simulink library "Course_Holes_Lib"  (R2026a)
settings: Solver=ode45  EnableMultiTasking=on
undefined symbols (not defined in the file): Mini_Golf_Param, X, Y, Z
libraries: Golf_Components_Lib x67, Contact_Forces_Lib x18, sm_lib x12
(part 2 of 2)

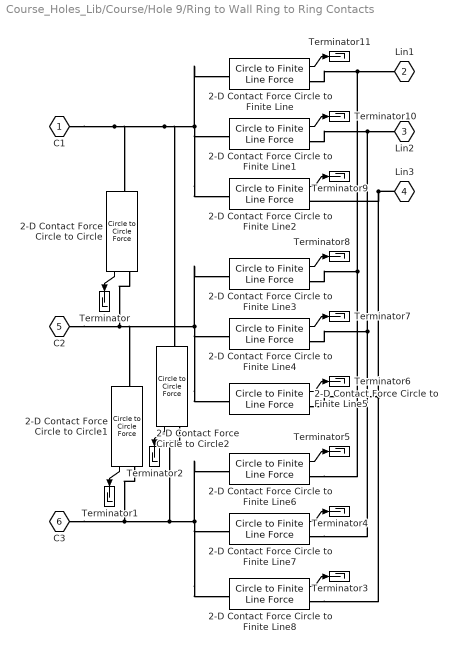
== system Course_Holes_Lib/Course/Hole 9/Ring to Wall Ring to Ring Contacts ==
  2-D Contact Force Circle to Circle : Contact_Forces_Lib/2D/Circle to Circle Force  cirB_rad=Mini_Golf_Param.Hole_9.Extr1.Ring_Outer_Diameter/2  cirF_rad=Mini_Golf_Param.Hole_9.Extr2.Ring_Outer_Diameter/2  active_angle=[-180 180]  force_law=Linear  k_contact=Mini_Golf_Param.Wall.Stiffness  b_contact=Mini_Golf_Param.Wall.Damping  pen_full_damp_F=1e-4  pen_exponent=1  custom_param_1=1  custom_param_2=1  friction_law=None  mu_kinetic=0.5  mu_static=0.7  v_thr=0.001  vis_on=off  vis_opc_en=0  vis_len_cirBz=0.1  vis_len_cirBx=0.005  vis_len_cirFz=0.1  vis_len_cirFx=0.005  vis_clr=[0.9 0.2 0.2]  vis_opc=0.7
      settings: SourceProductName=Simscape Multibody Contact Forces Library
  2-D Contact Force Circle to Circle1 : Contact_Forces_Lib/2D/Circle to Circle Force  cirB_rad=Mini_Golf_Param.Hole_9.Extr3.Ring_Outer_Diameter/2  cirF_rad=Mini_Golf_Param.Hole_9.Extr2.Ring_Outer_Diameter/2  active_angle=[-180 180]  force_law=Linear  k_contact=Mini_Golf_Param.Wall.Stiffness  b_contact=Mini_Golf_Param.Wall.Damping  pen_full_damp_F=1e-4  pen_exponent=1  custom_param_1=1  custom_param_2=1  friction_law=None  mu_kinetic=0.5  mu_static=0.7  v_thr=0.001  vis_on=off  vis_opc_en=0  vis_len_cirBz=0.1  vis_len_cirBx=0.005  vis_len_cirFz=0.1  vis_len_cirFx=0.005  vis_clr=[0.9 0.2 0.2]  vis_opc=0.7
      settings: SourceProductName=Simscape Multibody Contact Forces Library
  2-D Contact Force Circle to Circle2 : Contact_Forces_Lib/2D/Circle to Circle Force  cirB_rad=Mini_Golf_Param.Hole_9.Extr3.Ring_Outer_Diameter/2  cirF_rad=Mini_Golf_Param.Hole_9.Extr1.Ring_Outer_Diameter/2  active_angle=[-180 180]  force_law=Linear  k_contact=Mini_Golf_Param.Wall.Stiffness  b_contact=Mini_Golf_Param.Wall.Damping  pen_full_damp_F=1e-4  pen_exponent=1  custom_param_1=1  custom_param_2=1  friction_law=None  mu_kinetic=0.5  mu_static=0.7  v_thr=0.001  vis_on=off  vis_opc_en=0  vis_len_cirBz=0.1  vis_len_cirBx=0.005  vis_len_cirFz=0.1  vis_len_cirFx=0.005  vis_clr=[0.9 0.2 0.2]  vis_opc=0.7
      settings: SourceProductName=Simscape Multibody Contact Forces Library
  2-D Contact Force Circle to Finite Line : Contact_Forces_Lib/2D/Circle to Finite Line Force  circle_rad=Mini_Golf_Param.Hole_9.Extr1.Ring_Outer_Diameter/2  line_depth=Mini_Golf_Param.Wall.Width/2  line_length=Mini_Golf_Param.Hole_9.Wall_Right.Length  force_law=Linear  k_contact=Mini_Golf_Param.Wall.Stiffness  b_contact=Mini_Golf_Param.Wall.Damping  pen_full_damp_F=1e-4  pen_exponent=1  custom_param_1=1  custom_param_2=1  friction_law=None  mu_kinetic=0.5  mu_static=0.7  v_thr=0.001  vis_on=off  vis_opc_en=0  vis_len_linBz=0.1  vis_len_linBx=0.005  vis_len_cirFz=0.1  vis_len_cirFx=0.005  vis_clr=[0.9 0.2 0.2]  vis_opc=0.7
      settings: SourceProductName=Simscape Multibody Contact Forces Library
  2-D Contact Force Circle to Finite Line1 : Contact_Forces_Lib/2D/Circle to Finite Line Force  circle_rad=Mini_Golf_Param.Hole_9.Extr1.Ring_Outer_Diameter/2  line_depth=Mini_Golf_Param.Wall.Width/2  line_length=Mini_Golf_Param.Hole_9.Wall_Back.Length  force_law=Linear  k_contact=Mini_Golf_Param.Wall.Stiffness  b_contact=Mini_Golf_Param.Wall.Damping  pen_full_damp_F=1e-4  pen_exponent=1  custom_param_1=1  custom_param_2=1  friction_law=None  mu_kinetic=0.5  mu_static=0.7  v_thr=0.001  vis_on=off  vis_opc_en=0  vis_len_linBz=0.1  vis_len_linBx=0.005  vis_len_cirFz=0.1  vis_len_cirFx=0.005  vis_clr=[0.9 0.2 0.2]  vis_opc=0.7
      settings: SourceProductName=Simscape Multibody Contact Forces Library
  2-D Contact Force Circle to Finite Line2 : Contact_Forces_Lib/2D/Circle to Finite Line Force  circle_rad=Mini_Golf_Param.Hole_9.Extr1.Ring_Outer_Diameter/2  line_depth=Mini_Golf_Param.Wall.Width/2  line_length=Mini_Golf_Param.Hole_9.Wall_Right.Length  force_law=Linear  k_contact=Mini_Golf_Param.Wall.Stiffness  b_contact=Mini_Golf_Param.Wall.Damping  pen_full_damp_F=1e-4  pen_exponent=1  custom_param_1=1  custom_param_2=1  friction_law=None  mu_kinetic=0.5  mu_static=0.7  v_thr=0.001  vis_on=off  vis_opc_en=0  vis_len_linBz=0.1  vis_len_linBx=0.005  vis_len_cirFz=0.1  vis_len_cirFx=0.005  vis_clr=[0.9 0.2 0.2]  vis_opc=0.7
      settings: SourceProductName=Simscape Multibody Contact Forces Library
  2-D Contact Force Circle to Finite Line3 : Contact_Forces_Lib/2D/Circle to Finite Line Force  circle_rad=Mini_Golf_Param.Hole_9.Extr2.Ring_Outer_Diameter/2  line_depth=Mini_Golf_Param.Wall.Width/2  line_length=Mini_Golf_Param.Hole_9.Wall_Right.Length  force_law=Linear  k_contact=Mini_Golf_Param.Wall.Stiffness  b_contact=Mini_Golf_Param.Wall.Damping  pen_full_damp_F=1e-4  pen_exponent=1  custom_param_1=1  custom_param_2=1  friction_law=None  mu_kinetic=0.5  mu_static=0.7  v_thr=0.001  vis_on=off  vis_opc_en=0  vis_len_linBz=0.1  vis_len_linBx=0.005  vis_len_cirFz=0.1  vis_len_cirFx=0.005  vis_clr=[0.9 0.2 0.2]  vis_opc=0.7
      settings: SourceProductName=Simscape Multibody Contact Forces Library
  2-D Contact Force Circle to Finite Line4 : Contact_Forces_Lib/2D/Circle to Finite Line Force  circle_rad=Mini_Golf_Param.Hole_9.Extr2.Ring_Outer_Diameter/2  line_depth=Mini_Golf_Param.Wall.Width/2  line_length=Mini_Golf_Param.Hole_9.Wall_Back.Length  force_law=Linear  k_contact=Mini_Golf_Param.Wall.Stiffness  b_contact=Mini_Golf_Param.Wall.Damping  pen_full_damp_F=1e-4  pen_exponent=1  custom_param_1=1  custom_param_2=1  friction_law=None  mu_kinetic=0.5  mu_static=0.7  v_thr=0.001  vis_on=off  vis_opc_en=0  vis_len_linBz=0.1  vis_len_linBx=0.005  vis_len_cirFz=0.1  vis_len_cirFx=0.005  vis_clr=[0.9 0.2 0.2]  vis_opc=0.7
      settings: SourceProductName=Simscape Multibody Contact Forces Library
  2-D Contact Force Circle to Finite Line5 : Contact_Forces_Lib/2D/Circle to Finite Line Force  circle_rad=Mini_Golf_Param.Hole_9.Extr2.Ring_Outer_Diameter/2  line_depth=Mini_Golf_Param.Wall.Width/2  line_length=Mini_Golf_Param.Hole_9.Wall_Right.Length  force_law=Linear  k_contact=Mini_Golf_Param.Wall.Stiffness  b_contact=Mini_Golf_Param.Wall.Damping  pen_full_damp_F=1e-4  pen_exponent=1  custom_param_1=1  custom_param_2=1  friction_law=None  mu_kinetic=0.5  mu_static=0.7  v_thr=0.001  vis_on=off  vis_opc_en=0  vis_len_linBz=0.1  vis_len_linBx=0.005  vis_len_cirFz=0.1  vis_len_cirFx=0.005  vis_clr=[0.9 0.2 0.2]  vis_opc=0.7
      settings: SourceProductName=Simscape Multibody Contact Forces Library
  2-D Contact Force Circle to Finite Line6 : Contact_Forces_Lib/2D/Circle to Finite Line Force  circle_rad=Mini_Golf_Param.Hole_9.Extr3.Ring_Outer_Diameter/2  line_depth=Mini_Golf_Param.Wall.Width/2  line_length=Mini_Golf_Param.Hole_9.Wall_Right.Length  force_law=Linear  k_contact=Mini_Golf_Param.Wall.Stiffness  b_contact=Mini_Golf_Param.Wall.Damping  pen_full_damp_F=1e-4  pen_exponent=1  custom_param_1=1  custom_param_2=1  friction_law=None  mu_kinetic=0.5  mu_static=0.7  v_thr=0.001  vis_on=off  vis_opc_en=0  vis_len_linBz=0.1  vis_len_linBx=0.005  vis_len_cirFz=0.1  vis_len_cirFx=0.005  vis_clr=[0.9 0.2 0.2]  vis_opc=0.7
      settings: SourceProductName=Simscape Multibody Contact Forces Library
  2-D Contact Force Circle to Finite Line7 : Contact_Forces_Lib/2D/Circle to Finite Line Force  circle_rad=Mini_Golf_Param.Hole_9.Extr3.Ring_Outer_Diameter/2  line_depth=Mini_Golf_Param.Wall.Width/2  line_length=Mini_Golf_Param.Hole_9.Wall_Back.Length  force_law=Linear  k_contact=Mini_Golf_Param.Wall.Stiffness  b_contact=Mini_Golf_Param.Wall.Damping  pen_full_damp_F=1e-4  pen_exponent=1  custom_param_1=1  custom_param_2=1  friction_law=None  mu_kinetic=0.5  mu_static=0.7  v_thr=0.001  vis_on=off  vis_opc_en=0  vis_len_linBz=0.1  vis_len_linBx=0.005  vis_len_cirFz=0.1  vis_len_cirFx=0.005  vis_clr=[0.9 0.2 0.2]  vis_opc=0.7
      settings: SourceProductName=Simscape Multibody Contact Forces Library
  2-D Contact Force Circle to Finite Line8 : Contact_Forces_Lib/2D/Circle to Finite Line Force  circle_rad=Mini_Golf_Param.Hole_9.Extr3.Ring_Outer_Diameter/2  line_depth=Mini_Golf_Param.Wall.Width/2  line_length=Mini_Golf_Param.Hole_9.Wall_Right.Length  force_law=Linear  k_contact=Mini_Golf_Param.Wall.Stiffness  b_contact=Mini_Golf_Param.Wall.Damping  pen_full_damp_F=1e-4  pen_exponent=1  custom_param_1=1  custom_param_2=1  friction_law=None  mu_kinetic=0.5  mu_static=0.7  v_thr=0.001  vis_on=off  vis_opc_en=0  vis_len_linBz=0.1  vis_len_linBx=0.005  vis_len_cirFz=0.1  vis_len_cirFx=0.005  vis_clr=[0.9 0.2 0.2]  vis_opc=0.7
      settings: SourceProductName=Simscape Multibody Contact Forces Library
  Terminator{,1..11} (12 alike) : Terminator
  C1 : PMIOPort  Side=Left
  Lin1 : PMIOPort  Port=2  Side=Right
  Lin2 : PMIOPort  Port=3  Side=Right
  Lin3 : PMIOPort  Port=4  Side=Right
  C2 : PMIOPort  Port=5  Side=Left
  C3 : PMIOPort  Port=6  Side=Left
  wires:
  2-D Contact Force Circle to Circle/1 -> Terminator/1
  2-D Contact Force Circle to Circle1/1 -> Terminator1/1
  2-D Contact Force Circle to Circle2/1 -> Terminator2/1
  2-D Contact Force Circle to Finite Line8/1 -> Terminator3/1
  2-D Contact Force Circle to Finite Line7/1 -> Terminator4/1
  2-D Contact Force Circle to Finite Line6/1 -> Terminator5/1
  2-D Contact Force Circle to Finite Line5/1 -> Terminator6/1
  2-D Contact Force Circle to Finite Line4/1 -> Terminator7/1
  2-D Contact Force Circle to Finite Line3/1 -> Terminator8/1
  2-D Contact Force Circle to Finite Line2/1 -> Terminator9/1
  2-D Contact Force Circle to Finite Line1/1 -> Terminator10/1
  2-D Contact Force Circle to Finite Line/1 -> Terminator11/1
  connections:
  2-D Contact Force Circle to Finite Line5/RConn1 -- 2-D Contact Force Circle to Finite Line8/RConn1 -- 2-D Contact Force Circle to Finite Line2/RConn1 -- Lin3/RConn1
  2-D Contact Force Circle to Finite Line4/RConn1 -- 2-D Contact Force Circle to Finite Line7/RConn1 -- 2-D Contact Force Circle to Finite Line1/RConn1 -- Lin2/RConn1
  2-D Contact Force Circle to Finite Line3/RConn1 -- 2-D Contact Force Circle to Finite Line6/RConn1 -- 2-D Contact Force Circle to Finite Line/RConn1 -- Lin1/RConn1
  C1/RConn1 -- 2-D Contact Force Circle to Circle/LConn1 -- 2-D Contact Force Circle to Circle2/LConn1 -- 2-D Contact Force Circle to Finite Line2/LConn1 -- 2-D Contact Force Circle to Finite Line1/LConn1 -- 2-D Contact Force Circle to Finite Line/LConn1
  C2/RConn1 -- 2-D Contact Force Circle to Circle1/LConn1 -- 2-D Contact Force Circle to Finite Line3/LConn1 -- 2-D Contact Force Circle to Finite Line4/LConn1 -- 2-D Contact Force Circle to Finite Line5/LConn1 -- 2-D Contact Force Circle to Circle/RConn1
  C3/RConn1 -- 2-D Contact Force Circle to Circle1/RConn1 -- 2-D Contact Force Circle to Circle2/RConn1 -- 2-D Contact Force Circle to Finite Line6/LConn1 -- 2-D Contact Force Circle to Finite Line7/LConn1 -- 2-D Contact Force Circle to Finite Line8/LConn1
